simulink model "S_mixedm"  (Simulink 7.6)
settings: Solver=ode5  SolverMode=SingleTasking  StartTime=0.0  StopTime=10.0  FixedStep=.1  MaxStep=.1  RelTol=1e-3  AbsTol=1e-6
Description:
  | Multiple Sample Time Integrator + Zero-Order Hold + Unit Delay C-MEX S-function
settings Model: Creator=The MathWorks Inc.  LastModifiedBy=admin  ExtModeTrigMode=oneshot  ExtModeArmWhenConnect=off  ExtModeAutoUpdateStatusClock=off
settings DataIOCC: ExternalInput=[]  InitialState=[]  LimitDataPoints=off  TimeSaveName=t  OutputSaveName=y
settings OptimizationCC: BlockReduction=off  BooleanDataType=off  InitFltsAndDblsToZero=on
settings DebuggingCC: SaveWithParameterizedLinksMsg=none  SignalResolutionControl=TryResolveAllWithWarning  SolverPrmCheckMsg=none  InheritedTsInSrcMsg=none  MultiTaskDSMMsg=warning  MultiTaskCondExecSysMsg=none  IntegerOverflowMsg=none
settings HardwareCC: TargetUnknown=on
settings RTWCC: IncludeERTFirstTime=on
settings CodeAppCC: CustomSymbolStrFcn=$F$N$M
settings GRTTargetCC: TargetFcnLib=ansi_tfl_tmw.mat

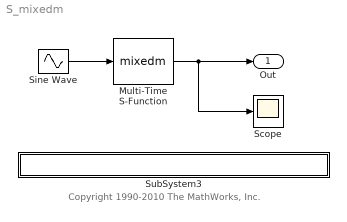
== system S_mixedm ==
  note: Copyright 1990-2010 The MathWorks, Inc.
  Multi-Time S-Function : S-Function  FunctionName=mixedm  EnableBusSupport=off
      mask Type: S-function: mixedm
      mask Description: This is a S-function that illustrates multiple sample time by implementing integrator -> ZOH(Ts=1second) -> UnitDelay(Ts=1second) with an initial condition of 1.
  Scope : Scope
      settings: TimeRange=10  YMin=1  YMax=3
  Sine Wave : Sin  SampleTime=0
  SubSystem3 : Subsystem  mask{filename=mixedm.c}
      mask init:
      | x=sfundemo_maskdisp;
      settings: AttributesFormatString=\n  OpenFcn=sfundemo_openfcn
      mask Display: disp(x);
  Out : Outport  InitialOutput=0
  wires:
  Sine Wave/1 -> Multi-Time S-Function/1
  Multi-Time S-Function/1 -> Out/1, Scope/1

== system S_mixedm/SubSystem3 ==
